simulink model "SPERTE_printer"  (R2026a)
settings: Solver=FixedStepDiscrete  StopTime=inf  FixedStep=Ts  EnableMultiTasking=on
InitFcn:
  | Fs = 1000; Ts = 1/Fs;tsim = Inf;
undefined symbols (not defined in the file or in its folder): DiscIntNeverNeededParam
libraries: simulink x11, sperte_lib x3
settings Model: SimulationMode=external  ExtModeTrigDuration=2  Creator=glife  LastModifiedBy=larsm
settings SolverCC: PositivePriorityOrder=on
settings OptimizationCC: PassReuseOutputArgsThreshold=0.0  MaxStackSize=200000
settings HardwareCC: ProdBitPerLong=64.0  ProdLargestAtomicInteger=LongLong  ProdLargestAtomicFloat=Double  ProdHWDeviceType=ARM Compatible->ARM Cortex-A (64-bit)  UseEmbeddedCoderFeatures=off
settings RTWCC: SystemTargetFile=ert.tlc  HardwareBoard=Raspberry Pi (64bit)  TLCOptions="-aInlineSetEventsForThisBaseRateFcn=TLC_FALSE -aSuppressMultiTaskScheduler=TLC_FALSE  -aRateBasedStepFcn=0"  PostCodeGenCommand="if (~verLessThan('matlab', '9.11')) codertarget.postCodeGenHookCommand(h);  SPERTE_postGenFunc(modelName, buildInfo); else; SPERTE_postGenFunc(h, buildInfo); end"  Toolchain=GNU GCC RPIUtils  BuildConfiguration=Faster Runs  Description=Embedded Coder
settings ERTTargetCC: ExtMode=on  ExtModeTransport=2.0  ExtModeMexArgs='131.155.56.35' 1 17725  ERTSrcFileBannerTemplate=codertarget_code_template.cgt  ERTHdrFileBannerTemplate=codertarget_code_template.cgt  ERTDataSrcFileTemplate=codertarget_code_template.cgt  ERTDataHdrFileTemplate=codertarget_code_template.cgt  DynamicArrayContainerType=coder::array  ERTCustomFileBanners=off  SupportContinuousTime=on  SupportNonInlinedSFcns=on  SupportVariableSizeSignals=on  ModelStepFunctionPrototypeControlCompliant=off

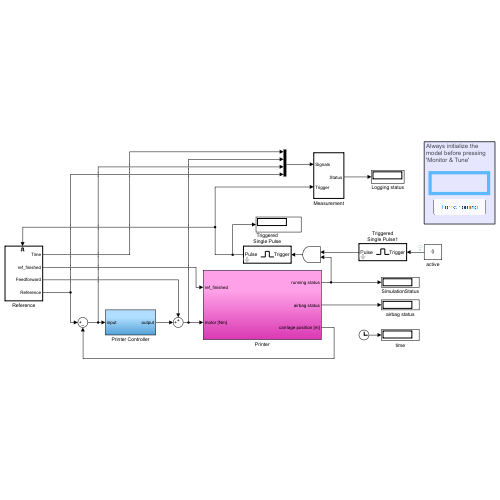
[thumbnail: Simulink's stored preview of the top-level diagram]
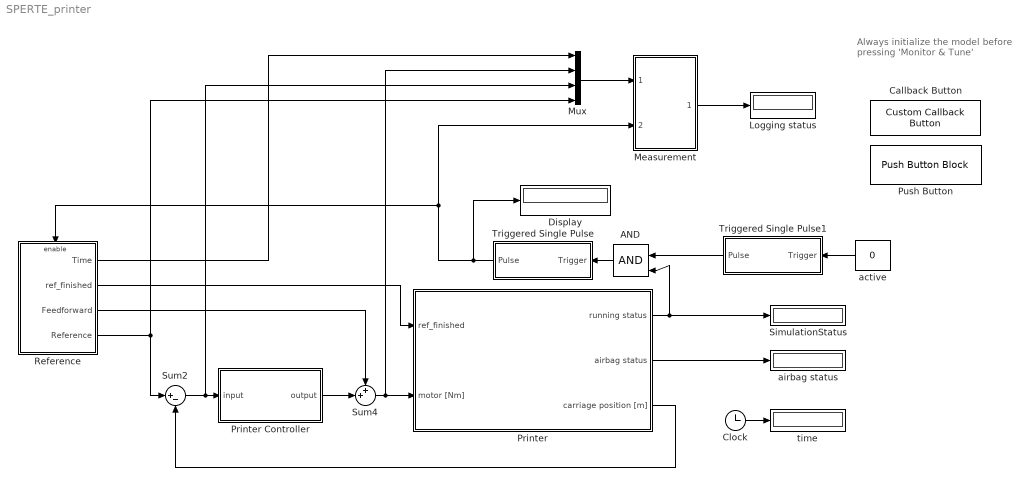
== system SPERTE_printer ==
  note: Always initialize the
      | model before pressing
      | 'Monitor & Tune'
  AND : Logic  IconShape=distinctive  AllPortsSameDT=off  OutDataTypeStr=boolean
  Callback Button : CustomCallbackButton  Configuration="{\"components\":[{\"name\":\"BackgroundImageComponent\",\"settings\":{\"image\":{\"size\":[0,0],\"src\":\"default\",\"srcOrientation\":\"Right\"},\"position\":[0,0,1,1]}},{\"name\":\"ButtonStateComponent\",\"settings\":{\"buttonType\":\"momentary\",\"clickFcn\":\"set_param('SPERTE_printer\\/Reference\\/set_Ref','Value','zeros(4501,1)');\\nset_param('SPERTE_printer\\/Reference\\/set_ff','Value','zeros(4501,1)');\\nset_param('SPERTE_printer\\/active','Value','0');\\nset_param('SPERTE_printer\\/Printer\\/force_home','Value','0');\\nmsgbox('Successfully initialized the model.');\",\"onValue\":1,\"position\":[0,0,1,1],\"pressDelay\":\"500\",\"pressFcn\":\"\",\"repeatInterval\":\"0\",\"states\":[{\"horizontalAlignment\":\"center\",\"image\":{\"position\":[0,0,1,1],\"src\":\"default\",\"srcOrientation\":\"Right\"},\"label\":{\"color\":[0.01176470588,0.01176470588,0.01176470588,1],\"icon\":{\"size\":[0,0],\"src\":\"default\",\"srcOrientation\":\"Right\"},\"iconPlacement\":\"left\",\"text\":{\"content\":\"INITIALIZE MODEL\"}},\"labelOffset\":[0,0],\"verticalAlignment\":\"middle\"},{\"horizontalAlignment\":\"center\",\"image\":{\"position\":[0,0,1,1],\"src\":\"default\",\"srcOrientation\":\"Right\"},\"label\":{\"color\":[0.01176470588,0.01176470588,0.01176470588,1],\"icon\":{\"size\":[0,0],\"src\":\"default\",\"srcOrientation\":\"Right\"},\"iconPlacement\":\"left\",\"text\":{\"content\":\"INITIALIZE MODEL\"}},\"labelOffset\":[0,0],\"verticalAlignment\":\"middle\"},{\"horizontalAlignment\":\"center\",\"image\":{\"position\":[0,0,1,1],\"src\":\"default\",\"srcOrientation\":\"Right\"},\"label\":{\"color\":[0.01176470588,0.01176470588,0.01176470588,1],\"icon\":{\"size\":[0,0],\"src\":\"default\",\"srcOrientation\":\"Right\"},\"iconPlacement\":\"left\",\"text\":{\"content\":\"INITIALIZE MODEL\"}},\"labelOffset\":[0,0],\"verticalAlignment\":\"middle\"},{\"horizontalAlignment\":\"center\",\"image\":{\"position\":[0,0,1,1],\"src\":\"default\",\"srcOrientation\":\"Right\"},\"label\":{\"color\":[0.01176470588,0.01176470588,0.01176470588,1],\"icon\":{\"size\":[0,0],\"src\":\"default\",\"srcOrientation\":\"Right\"},\"iconPlacement\":\"left\",\"text\":{\"content\":\"INITIALIZE MODEL\"}},\"labelOffset\":[0,0],\"verticalAlignment\":\"middle\"}]}},{\"name\":\"ForegroundImageComponent\",\"settings\":{\"image\":{\"size\":[0,0],\"src\":\"default\",\"srcOrientation\":\"Right\"},\"isForeground\":1,\"position\":[0,0,1,1]}}],\"derived\":{\"blockParameters\":{\"AutoActivate\":true,\"ButtonText\":\"INITIALIZE MODEL\",\"ButtonType\":\"Momentary\",\"ClickFcn\":\"set_param('SPERTE_printer\\/Reference\\/set_Ref','Value','zeros(4501,1)');\\nset_param('SPERTE_printer\\/Reference\\/set_ff','Value','zeros(4501,1)');\\nset_param('SPERTE_printer\\/active','Value','0');\\nset_param('SPERTE_printer\\/Printer\\/force_home','Value','0');\\nmsgbox('Successfully initialized the model.');\",\"OnValue\":1,\"PressDelay\":\"500\",\"PressFcn\":\"\",\"RepeatInterval\":\"0\",\"fixedAspectRatio\":\"off\"}},\"settings\":{\"BindingType\":\"standalone\",\"autoActivate\":true,\"backgroundColor\":[244,244,244,1],\"backgroundOffset\":0.2,\"backgroundOpacity\":1,\"fixedAspectRatio\":\"off\",\"foregroundColor\":[0.01176470588,0.01176470588,0.01176470588,1],\"migratedFromLegacy\":true,\"useBackgroundColor\":true,\"variant\":\"callback\",\"version\":\"R2024b\"},\"type\":\"Button\"}"  CustomBackgroundColor="{\"color\":[0.9568627451,0.9568627451,0.9568627451],\"show\":true}"
  Clock : Clock
  Display : Display
  Logging status : Display
  Measurement : Subsystem  TreatAsAtomicUnit=on
  Mux : Mux
  Printer : Subsystem
  Printer Controller : Subsystem
  Push Button : PushButtonBlock  ButtonText=Force homing  IconOnColor=[0.0, 0.39215686274509803, 0.0]  IconOffColor=[0.0, 1.0, 0.0]  OffValue=0.000000
  Reference : Subsystem  TreatAsAtomicUnit=on
  SimulationStatus : Display
      settings: Decimation=50
  Sum2 : Sum  Inputs=|+-
  Sum4 : Sum  Inputs=++|  InputSameDT=on  SaturateOnIntegerOverflow=on  OutDataTypeStr=Inherit: Same as first input
  Triggered Single Pulse : Subsystem  TreatAsAtomicUnit=on  mask(single pulse generation){p_wid=4502}
      mask prompts: p_wid "pulse width (number of samples)"
      mask help: This block generate a single pulse whenever a trigger happen. The pulse width must specified as a number of samples. for example if your sampling time is 0.1s and you want 3s pulse , then you should enter 30 as a pulse width.
      mask Display:
      | plot([0],[0])
      | plot([11],[0])
      | plot([5],[0.5])
      | plot([4 5 5 6 6 7],[0 0 0.25 0.25 0 0])
      | plot([5],[-0.3])
      | 
      | port_label('output', 1, 'Pulse')
      | port_label('input', 1, 'Trigger')
  Triggered Single Pulse1 : Subsystem  TreatAsAtomicUnit=on  mask(single pulse generation){p_wid=4502}
      mask prompts: p_wid "pulse width (number of samples)"
      mask help: This block generate a single pulse whenever a trigger happen. The pulse width must specified as a number of samples. for example if your sampling time is 0.1s and you want 3s pulse , then you should enter 30 as a pulse width.
      mask Display:
      | plot([0],[0])
      | plot([11],[0])
      | plot([5],[0.5])
      | plot([4 5 5 6 6 7],[0 0 0.25 0.25 0 0])
      | plot([5],[-0.3])
      | 
      | port_label('output', 1, 'Pulse')
      | port_label('input', 1, 'Trigger')
  active : Constant  Value=0
  airbag status : Display
      settings: Decimation=50
  time : Display
      settings: Decimation=50
  wires:
  Printer/3(carriage position [m]) -> Sum2/2
  Printer/2(airbag status) -> airbag status/1
  Sum2/1 -> Printer Controller/1(input), Mux/3
  Sum4/1 -> Printer/2(motor [Nm]), Mux/2
  Clock/1 -> time/1
  Printer Controller/1(output) -> Sum4/2
  AND/1 -> Triggered Single Pulse/1(Trigger)
  Reference/4(Reference) -> Sum2/1, Mux/4
  Reference/1(Time) -> Mux/1
  Mux/1 -> Measurement/1(Signals)
  Measurement/1(Status) -> Logging status/1
  Reference/3(Feedforward) -> Sum4/1
  Reference/2(ref_finished) -> Printer/1(ref_finished)
  Printer/1(running status) -> SimulationStatus/1, AND/2
  active/1 -> Triggered Single Pulse1/1(Trigger)
  Triggered Single Pulse/1(Pulse) -> Display/1, Measurement/2(Trigger), Reference/Enable
  Triggered Single Pulse1/1(Pulse) -> AND/1

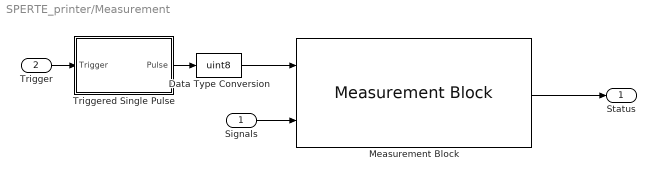
== system SPERTE_printer/Measurement ==
  Signals : Inport
  Trigger : Inport  Port=2
  Data Type Conversion : DataTypeConversion  OutDataTypeStr=uint8  SaturateOnIntegerOverflow=off  RndMeth=Floor
  Measurement Block : sperte_lib/Measurement/Measurement Block  Description=|  Priority=-1  N_samples=4501  triggertype=2  trigger_command=0
      | Perform on-demand measurements to file using this block.
      | 
      | It can be used in 2 ways:
      | 1) Set the mask triggertype parameter to manual and use the trigger input signal to trigger a measurement.
      | You can do this by providing a 0 to 1 transition.
      | Keep it low after you start/complete the measurement, or it will measure again.
      | A file is created with measurement_0,1,2... etc
      | 
      | 2) Keep the model running, and trigger a measurement from the commandline or Matlab script.
      | For example:
      | 
      | % How many samples to measure?
      | N_samples = Fs*5;
      | % Do the measurement
      | SPERTE_Perform_Measurement(N_samples);
      | % Get the latest file
      | file_list = SPERTE_Get_Latest_Measurement(p,1,'./data');
      | % How many signals did you record?
      | N_signals = 3;
      | % Convert the .bin to .mat and return the results
      | measurement = SPERTE_Bin_To_Mat(file_list,N_signals);
      settings: SourceProductName=SPERTE library
  Triggered Single Pulse : Subsystem  TreatAsAtomicUnit=on  mask(single pulse generation){p_wid=20}
      mask prompts: p_wid "pulse width (number of samples)"
      mask help: This block generate a single pulse whenever a trigger happen. The pulse width must specified as a number of samples. for example if your sampling time is 0.1s and you want 3s pulse , then you should enter 30 as a pulse width.
      mask Display:
      | plot([0],[0])
      | plot([11],[0])
      | plot([5],[0.5])
      | plot([4 5 5 6 6 7],[0 0 0.25 0.25 0 0])
      | plot([5],[-0.3])
      | 
      | port_label('output', 1, 'Pulse')
      | port_label('input', 1, 'Trigger')
  Status : Outport
  wires:
  Data Type Conversion/1 -> Measurement Block/1
  Measurement Block/1 -> Status/1
  Signals/1 -> Measurement Block/2
  Triggered Single Pulse/1(Pulse) -> Data Type Conversion/1
  Trigger/1 -> Triggered Single Pulse/1(Trigger)

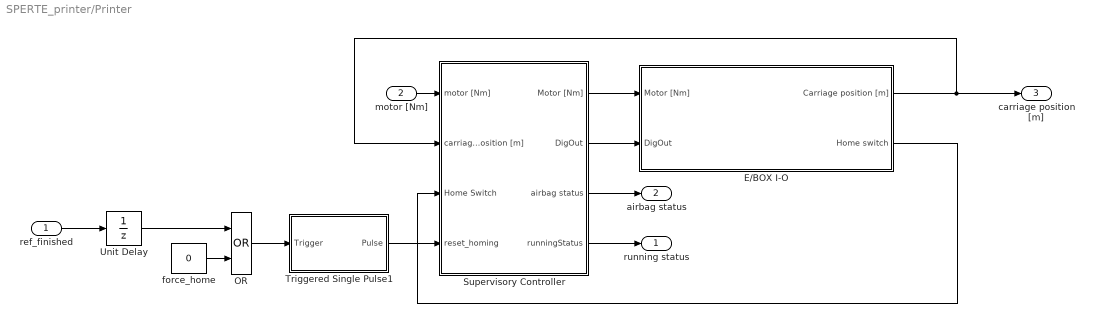
== system SPERTE_printer/Printer ==
  ref_finished : Inport
  motor [Nm] : Inport  Port=2
  E/BOX I-O : Subsystem
  OR : Logic  Operator=OR  IconShape=distinctive  AllPortsSameDT=off  OutDataTypeStr=boolean
  Supervisory Controller : Subsystem
  Triggered Single Pulse1 : Subsystem  TreatAsAtomicUnit=on  mask(single pulse generation){p_wid=1}
      mask prompts: p_wid "pulse width (number of samples)"
      mask help: This block generate a single pulse whenever a trigger happen. The pulse width must specified as a number of samples. for example if your sampling time is 0.1s and you want 3s pulse , then you should enter 30 as a pulse width.
      mask Display:
      | plot([0],[0])
      | plot([11],[0])
      | plot([5],[0.5])
      | plot([4 5 5 6 6 7],[0 0 0.25 0.25 0 0])
      | plot([5],[-0.3])
      | 
      | port_label('output', 1, 'Pulse')
      | port_label('input', 1, 'Trigger')
  Unit Delay : UnitDelay  SampleTime=-1
  force_home : Constant  Value=0
  running status : Outport
  airbag status : Outport  Port=2
  carriage position [m] : Outport  Port=3
  wires:
  E/BOX I-O/1(Carriage position [m]) -> Supervisory Controller/2(carriage position [m]), carriage position [m]/1
  Supervisory Controller/1(Motor [Nm]) -> E/BOX I-O/1(Motor [Nm])
  E/BOX I-O/2(Home switch) -> Supervisory Controller/3(Home Switch)
  motor [Nm]/1 -> Supervisory Controller/1(motor [Nm])
  Supervisory Controller/3(airbag status) -> airbag status/1
  Supervisory Controller/4(runningStatus) -> running status/1
  Supervisory Controller/2(DigOut) -> E/BOX I-O/2(DigOut)
  ref_finished/1 -> Unit Delay/1
  Triggered Single Pulse1/1(Pulse) -> Supervisory Controller/4(reset_homing)
  OR/1 -> Triggered Single Pulse1/1(Trigger)
  force_home/1 -> OR/2
  Unit Delay/1 -> OR/1

== system SPERTE_printer/Printer Controller ==
  input : Inport
  Dct2lowpass : S-Function  FunctionName=dlowpass2  Parameters=f_den, b_den, 0.001  SFunctionDeploymentMode=off  EnableBusSupport=off  mask(dctools){f_den=40, b_den=0.7}
      mask prompts: f_den "Pole [Hz]"; b_den "Damping pole [-]"
      mask help: This block implements a discrete time 2nd order lowpass filter.
      mask Display: disp('DCT 2nd order lowpass')
  Dctpd : S-Function  FunctionName=dpd  Parameters=kp, kv, 0.001  SFunctionDeploymentMode=off  EnableBusSupport=off  mask(dctools){kp=40, kv=1}
      mask help: This block implements a discrete time pd filter.
      mask Display: disp('DCT pd')
  Gain : Gain  Gain=4  SaturateOnIntegerOverflow=on  OutDataTypeStr=Inherit: Same as input  ParamDataTypeStr=Inherit: Same as input
  output : Outport
  wires:
  input/1 -> Gain/1
  Gain/1 -> Dctpd/1
  Dctpd/1 -> Dct2lowpass/1
  Dct2lowpass/1 -> output/1

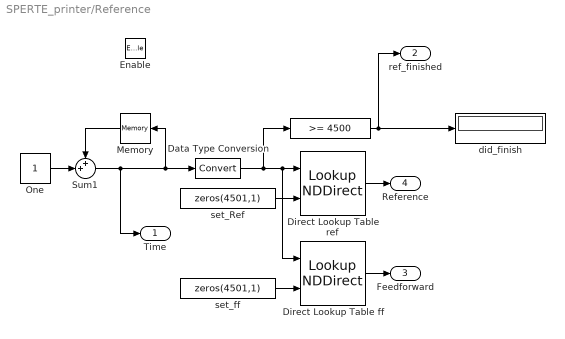
== system SPERTE_printer/Reference ==
  Enable : EnablePort  StatesWhenEnabling=reset
  " " : simulink/Logic and Bit Operations/Compare To Constant  relop=>=  const=4500  OutDataTypeStr=boolean
  Data Type Conversion : DataTypeConversion  SaturateOnIntegerOverflow=off  RndMeth=Floor
  Direct Lookup Table ff : LookupNDDirect  NumberOfTableDimensions=1  TableIsInput=on  Table=[4 5 ;16 19 ]  DiagnosticForOutOfRangeInput=Error
  Direct Lookup Table ref : LookupNDDirect  NumberOfTableDimensions=1  TableIsInput=on  Table=[4 5 ;16 19 ]  DiagnosticForOutOfRangeInput=Error
  Memory : Memory
  One : Constant  OutDataTypeStr=Inherit: Inherit via back propagation
  Sum1 : Sum  Inputs=++|
  did_finish : Display
  set_Ref : Constant  Value=zeros(4501,1)
  set_ff : Constant  Value=zeros(4501,1)
  Time : Outport
  ref_finished : Outport  Port=2
  Feedforward : Outport  Port=3
  Reference : Outport  Port=4
  wires:
  set_Ref/1 -> Direct Lookup Table ref/2
  Data Type Conversion/1 -> Direct Lookup Table ff/1, Direct Lookup Table ref/1, " "/1
  One/1 -> Sum1/2
  Direct Lookup Table ref/1 -> Reference/1
  Sum1/1 -> Data Type Conversion/1, Memory/1, Time/1
  Memory/1 -> Sum1/1
  Direct Lookup Table ff/1 -> Feedforward/1
  set_ff/1 -> Direct Lookup Table ff/2
  " "/1 -> did_finish/1, ref_finished/1

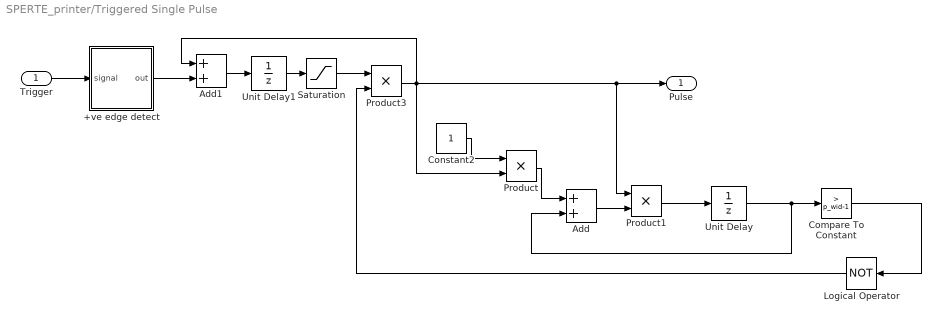
== system SPERTE_printer/Triggered Single Pulse ==
  Trigger : Inport
  +ve edge detect : Subsystem
  Add : Sum
  Add1 : Sum
  Compare To Constant : simulink/Logic and Bit Operations/Compare To Constant  relop=>  const=p_wid-1  OutDataTypeStr=boolean
  Constant2 : Constant
  Logical Operator : Logic  Operator=NOT  AllPortsSameDT=off  OutDataTypeStr=boolean
  Product : Product  RndMeth=Zero
  Product1 : Product  RndMeth=Zero
  Product3 : Product  RndMeth=Zero
  Saturation : Saturate  UpperLimit=1  LowerLimit=0
  Unit Delay : UnitDelay  SampleTime=-1
  Unit Delay1 : UnitDelay  SampleTime=-1
  Pulse : Outport
  wires:
  Compare To Constant/1 -> Logical Operator/1
  Constant2/1 -> Product/1
  Product/1 -> Add/1
  Unit Delay/1 -> Add/2, Compare To Constant/1
  Trigger/1 -> +ve edge detect/1(signal)
  +ve edge detect/1(out) -> Add1/2
  Add/1 -> Product1/2
  Product1/1 -> Unit Delay/1
  Add1/1 -> Unit Delay1/1
  Unit Delay1/1 -> Saturation/1
  Saturation/1 -> Product3/1
  Product3/1 -> Add1/1, Product/2, Product1/1, Pulse/1
  Logical Operator/1 -> Product3/2

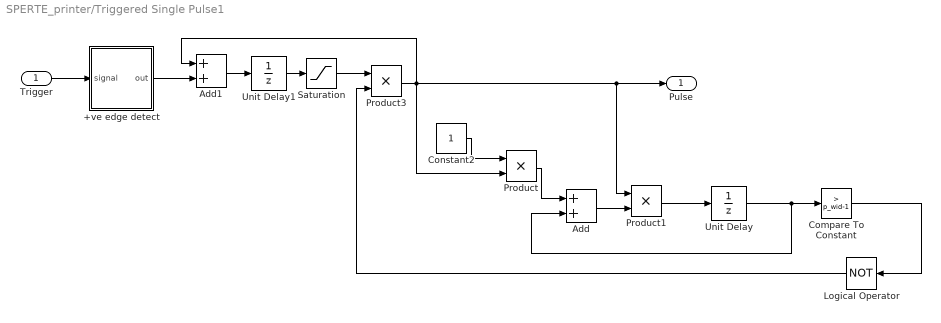
== system SPERTE_printer/Triggered Single Pulse1 ==
  Trigger : Inport
  +ve edge detect : Subsystem
  Add : Sum
  Add1 : Sum
  Compare To Constant : simulink/Logic and Bit Operations/Compare To Constant  relop=>  const=p_wid-1  OutDataTypeStr=boolean
  Constant2 : Constant
  Logical Operator : Logic  Operator=NOT  AllPortsSameDT=off  OutDataTypeStr=boolean
  Product : Product  RndMeth=Zero
  Product1 : Product  RndMeth=Zero
  Product3 : Product  RndMeth=Zero
  Saturation : Saturate  UpperLimit=1  LowerLimit=0
  Unit Delay : UnitDelay  SampleTime=-1
  Unit Delay1 : UnitDelay  SampleTime=-1
  Pulse : Outport
  wires:
  Compare To Constant/1 -> Logical Operator/1
  Constant2/1 -> Product/1
  Product/1 -> Add/1
  Unit Delay/1 -> Add/2, Compare To Constant/1
  Trigger/1 -> +ve edge detect/1(signal)
  +ve edge detect/1(out) -> Add1/2
  Add/1 -> Product1/2
  Product1/1 -> Unit Delay/1
  Add1/1 -> Unit Delay1/1
  Unit Delay1/1 -> Saturation/1
  Saturation/1 -> Product3/1
  Product3/1 -> Add1/1, Product/2, Product1/1, Pulse/1
  Logical Operator/1 -> Product3/2

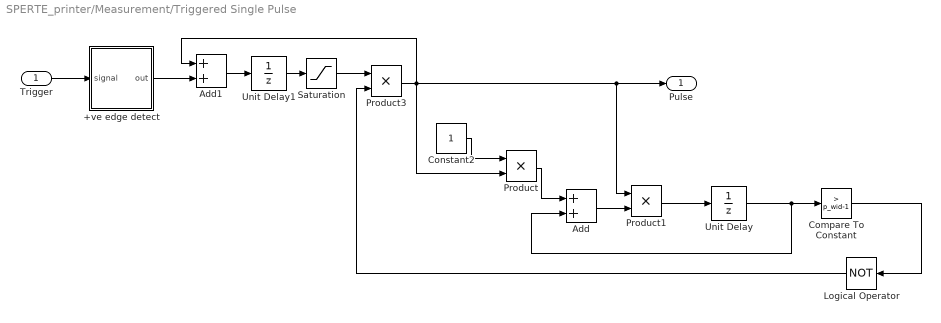
== system SPERTE_printer/Measurement/Triggered Single Pulse ==
  Trigger : Inport
  +ve edge detect : Subsystem
  Add : Sum
  Add1 : Sum
  Compare To Constant : simulink/Logic and Bit Operations/Compare To Constant  relop=>  const=p_wid-1  OutDataTypeStr=boolean
  Constant2 : Constant
  Logical Operator : Logic  Operator=NOT  AllPortsSameDT=off  OutDataTypeStr=boolean
  Product : Product  RndMeth=Zero
  Product1 : Product  RndMeth=Zero
  Product3 : Product  RndMeth=Zero
  Saturation : Saturate  UpperLimit=1  LowerLimit=0
  Unit Delay : UnitDelay  SampleTime=-1
  Unit Delay1 : UnitDelay  SampleTime=-1
  Pulse : Outport
  wires:
  Compare To Constant/1 -> Logical Operator/1
  Constant2/1 -> Product/1
  Product/1 -> Add/1
  Unit Delay/1 -> Add/2, Compare To Constant/1
  Trigger/1 -> +ve edge detect/1(signal)
  +ve edge detect/1(out) -> Add1/2
  Add/1 -> Product1/2
  Product1/1 -> Unit Delay/1
  Add1/1 -> Unit Delay1/1
  Unit Delay1/1 -> Saturation/1
  Saturation/1 -> Product3/1
  Product3/1 -> Add1/1, Product/2, Product1/1, Pulse/1
  Logical Operator/1 -> Product3/2

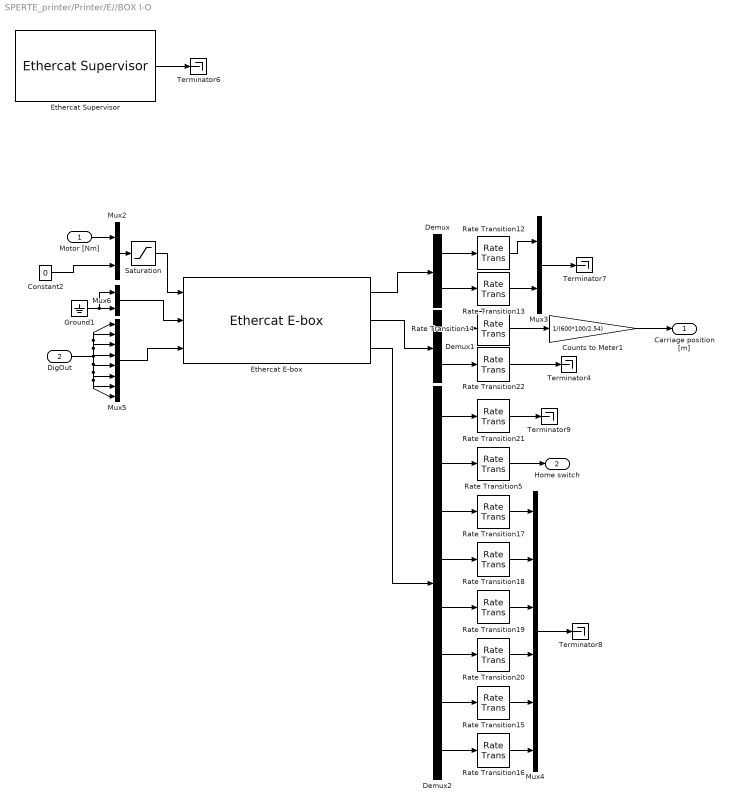
== system SPERTE_printer/Printer/E//BOX I-O ==
  Motor [Nm] : Inport
  DigOut : Inport  Port=2
  Constant2 : Constant  Value=0
  Counts to Meter1 : Gain  Gain=1/(600*100/2.54)
  Demux : Demux  Outputs=2
  Demux1 : Demux  Outputs=2
  Demux2 : Demux  Outputs=8
  Ethercat E-box : sperte_lib/EtherCAT/Ethercat E-box  Priority=-2  link_id=0
      settings: SourceProductName=SPERTE library
  Ethercat Supervisor : sperte_lib/EtherCAT/Ethercat Supervisor  Description=Must be executed first, keep at -1 priority (highest)  Priority=-3  portid=0  ectimeout=500
      settings: SourceProductName=SPERTE library
  Ground1 : Ground
  Mux2 : Mux  Inputs=2
  Mux3 : Mux  Inputs=2
  Mux4 : Mux  Inputs=6
  Mux5 : Mux  Inputs=8
  Mux6 : Mux  Inputs=2
  Rate Transition{5,12..22} (12 alike) : RateTransition
  Saturation : Saturate  UpperLimit=2.5  LowerLimit=-2.5
  Terminator{4,6..9} (5 alike) : Terminator
  Carriage position [m] : Outport
  Home switch : Outport  Port=2
  wires:
  Motor [Nm]/1 -> Mux2/1
  Demux2/2 -> Rate Transition5/1
  Rate Transition5/1 -> Home switch/1
  Saturation/1 -> Ethercat E-box/1
  Ethercat E-box/3 -> Demux2/1
  Ground1/1 -> Mux6/1, Mux6/2
  Ethercat Supervisor/1 -> Terminator6/1
  Ethercat E-box/2 -> Demux1/1
  Constant2/1 -> Mux2/2
  Mux2/1 -> Saturation/1
  Counts to Meter1/1 -> Carriage position [m]/1
  Ethercat E-box/1 -> Demux/1
  Demux/1 -> Rate Transition12/1
  Demux/2 -> Rate Transition13/1
  Rate Transition13/1 -> Mux3/2
  Mux3/1 -> Terminator7/1
  Rate Transition12/1 -> Mux3/1
  Rate Transition14/1 -> Counts to Meter1/1
  Demux1/1 -> Rate Transition14/1
  Demux1/2 -> Rate Transition22/1
  Rate Transition19/1 -> Mux4/3
  Rate Transition18/1 -> Mux4/2
  Rate Transition20/1 -> Mux4/4
  Demux2/8 -> Rate Transition16/1
  Rate Transition17/1 -> Mux4/1
  Demux2/5 -> Rate Transition19/1
  Demux2/6 -> Rate Transition20/1
  Demux2/4 -> Rate Transition18/1
  Rate Transition15/1 -> Mux4/5
  Mux4/1 -> Terminator8/1
  Demux2/3 -> Rate Transition17/1
  Demux2/7 -> Rate Transition15/1
  Rate Transition16/1 -> Mux4/6
  Rate Transition21/1 -> Terminator9/1
  Demux2/1 -> Rate Transition21/1
  Mux5/1 -> Ethercat E-box/3
  DigOut/1 -> Mux5/8, Mux5/7, Mux5/6, Mux5/5, Mux5/4, Mux5/1, Mux5/2, Mux5/3
  Mux6/1 -> Ethercat E-box/2
  Rate Transition22/1 -> Terminator4/1

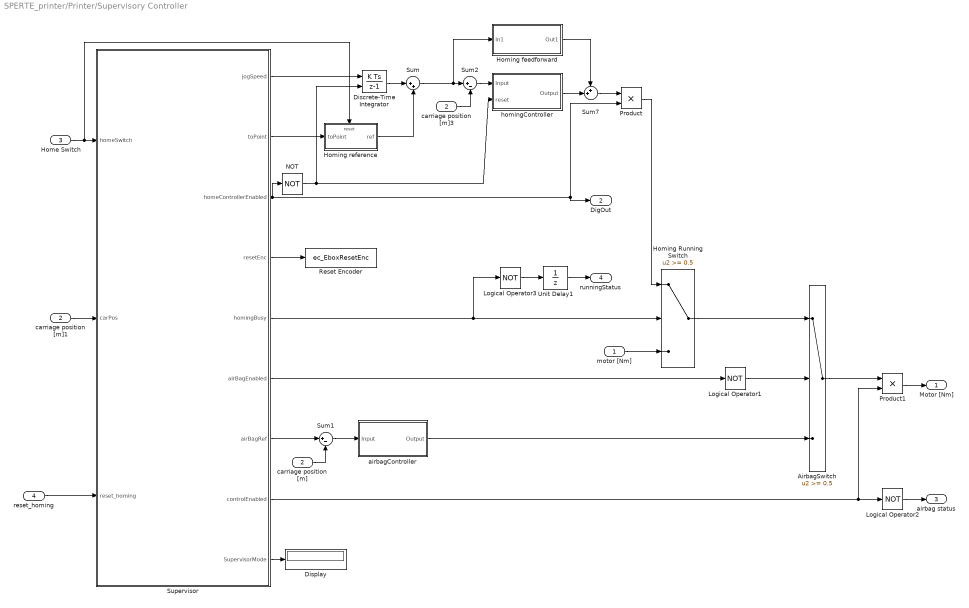
== system SPERTE_printer/Printer/Supervisory Controller ==
  motor [Nm] : Inport
  carriage position [m] : Inport  Port=2
  Home Switch : Inport  Port=3
  reset_homing : Inport  Port=4
  AirbagSwitch : Switch  Threshold=0.5  SaturateOnIntegerOverflow=off  InputSameDT=off
  Discrete-Time Integrator : DiscreteIntegrator  ExternalReset=level  SampleTime=-1  ICPrevOutput=DiscIntNeverNeededParam  ICPrevScaledInput=DiscIntNeverNeededParam
  Display : Display
  Homing Running Switch : Switch  Threshold=0.5  SaturateOnIntegerOverflow=off  InputSameDT=off
  Homing feedforward : Subsystem
  Homing reference : Subsystem
  Logical Operator1 : Logic  Operator=NOT  AllPortsSameDT=off  OutDataTypeStr=boolean
  Logical Operator2 : Logic  Operator=NOT  AllPortsSameDT=off  OutDataTypeStr=boolean
  Logical Operator3 : Logic  Operator=NOT  AllPortsSameDT=off  OutDataTypeStr=boolean
  NOT : Logic  Operator=NOT  IconShape=distinctive  AllPortsSameDT=off  OutDataTypeStr=boolean
  Product : Product  RndMeth=Zero
  Product1 : Product  RndMeth=Zero
  Reset Encoder : S-Function  FunctionName=ec_EboxResetEnc  Parameters=link_id  SFunctionDeploymentMode=off  EnableBusSupport=off  mask{link_id=0}
      mask prompts: link_id "analog in id (start from 1)"
  Sum : Sum  Inputs=|++
  Sum1 : Sum  Inputs=|+-
  Sum2 : Sum  Inputs=|+-
  Sum7 : Sum  Inputs=++|
  Supervisor : Stateflow chart  TreatAsAtomicUnit=on
  Unit Delay1 : UnitDelay  SampleTime=-1
  airbagController : Subsystem
  carriage position [m]1 : InportShadow  Port=2
  carriage position [m]3 : InportShadow  Port=2
  homingController : Subsystem
  Motor [Nm] : Outport
  DigOut : Outport  Port=2
  airbag status : Outport  Port=3
  runningStatus : Outport  Port=4
  wires:
  Homing Running Switch/1 -> AirbagSwitch/1
  Sum/1 -> Homing feedforward/1(In1), Sum2/1
  Sum2/1 -> homingController/1(Input)
  Home Switch/1 -> Homing reference/Reset, Supervisor/1(homeSwitch)
  Supervisor/1(jogSpeed) -> Discrete-Time Integrator/1
  carriage position [m]3/1 -> Sum2/2
  motor [Nm]/1 -> Homing Running Switch/3
  homingController/1(Output) -> Sum7/2
  Product/1 -> Homing Running Switch/1
  Discrete-Time Integrator/1 -> Sum/1
  Supervisor/5(homingBusy) -> Homing Running Switch/2, Logical Operator3/1
  Supervisor/3(homeControllerEnabled) -> Product/2, DigOut/1, NOT/1
  Supervisor/2(toPoint) -> Homing reference/1(toPoint)
  Supervisor/4(resetEnc) -> Reset Encoder/1
  carriage position [m]1/1 -> Supervisor/2(carPos)
  Supervisor/6(airBagEnabled) -> Logical Operator1/1
  Logical Operator1/1 -> AirbagSwitch/2
  airbagController/1(Output) -> AirbagSwitch/3
  Sum1/1 -> airbagController/1(Input)
  carriage position [m]/1 -> Sum1/2
  Supervisor/7(airBagRef) -> Sum1/1
  AirbagSwitch/1 -> Product1/1
  Product1/1 -> Motor [Nm]/1
  Supervisor/8(controlEnabled) -> Logical Operator2/1, Product1/2
  Logical Operator2/1 -> airbag status/1
  Logical Operator3/1 -> Unit Delay1/1
  Supervisor/9(SupervisorMode) -> Display/1
  Unit Delay1/1 -> runningStatus/1
  reset_homing/1 -> Supervisor/3(reset_homing)
  NOT/1 -> homingController/2(reset), Discrete-Time Integrator/2
  Sum7/1 -> Product/1
  Homing reference/1(ref) -> Sum/2
  Homing feedforward/1(Out1) -> Sum7/1

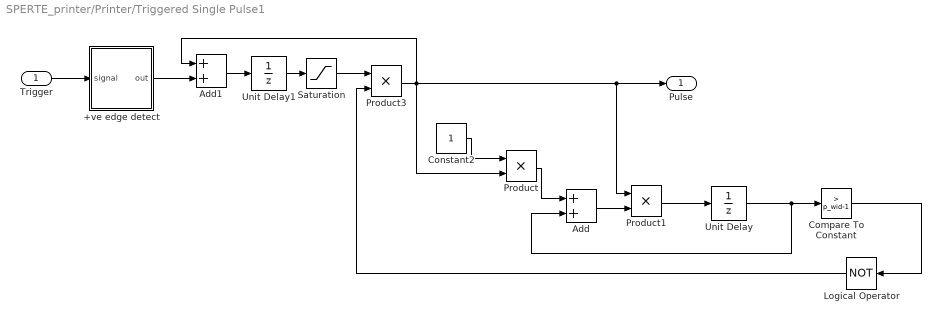
== system SPERTE_printer/Printer/Triggered Single Pulse1 ==
  Trigger : Inport
  +ve edge detect : Subsystem
  Add : Sum
  Add1 : Sum
  Compare To Constant : simulink/Logic and Bit Operations/Compare To Constant  relop=>  const=p_wid-1  OutDataTypeStr=boolean
  Constant2 : Constant
  Logical Operator : Logic  Operator=NOT  AllPortsSameDT=off  OutDataTypeStr=boolean
  Product : Product  RndMeth=Zero
  Product1 : Product  RndMeth=Zero
  Product3 : Product  RndMeth=Zero
  Saturation : Saturate  UpperLimit=1  LowerLimit=0
  Unit Delay : UnitDelay  SampleTime=-1
  Unit Delay1 : UnitDelay  SampleTime=-1
  Pulse : Outport
  wires:
  Compare To Constant/1 -> Logical Operator/1
  Constant2/1 -> Product/1
  Product/1 -> Add/1
  Unit Delay/1 -> Add/2, Compare To Constant/1
  Trigger/1 -> +ve edge detect/1(signal)
  +ve edge detect/1(out) -> Add1/2
  Add/1 -> Product1/2
  Product1/1 -> Unit Delay/1
  Add1/1 -> Unit Delay1/1
  Unit Delay1/1 -> Saturation/1
  Saturation/1 -> Product3/1
  Product3/1 -> Add1/1, Product/2, Product1/1, Pulse/1
  Logical Operator/1 -> Product3/2

== system SPERTE_printer/Triggered Single Pulse/+ve edge detect ==
  note: Edge
  signal : Inport
  Delay Input1 : UnitDelay  Description=Store in Global RAM  DisableCoverage=on  SampleTime=-1
  FixPt Relational Operator : RelationalOperator  Operator=>  OutDataTypeStr=fixdt(0, 8)  ZeroCross=off  InputSameDT=off
  Positive : simulink/Logic and Bit Operations/Compare To Zero  relop=>  OutDataTypeStr=uint8  ZeroCross=off
  out : Outport
  wires:
  Delay Input1/1 -> FixPt Relational Operator/2  "U(k-1)"
  Positive/1 -> Delay Input1/1, FixPt Relational Operator/1  "U(k)"
  FixPt Relational Operator/1 -> out/1
  signal/1 -> Positive/1

== system SPERTE_printer/Triggered Single Pulse1/+ve edge detect ==
  note: Edge
  signal : Inport
  Delay Input1 : UnitDelay  Description=Store in Global RAM  DisableCoverage=on  SampleTime=-1
  FixPt Relational Operator : RelationalOperator  Operator=>  OutDataTypeStr=fixdt(0, 8)  ZeroCross=off  InputSameDT=off
  Positive : simulink/Logic and Bit Operations/Compare To Zero  relop=>  OutDataTypeStr=uint8  ZeroCross=off
  out : Outport
  wires:
  Delay Input1/1 -> FixPt Relational Operator/2  "U(k-1)"
  Positive/1 -> Delay Input1/1, FixPt Relational Operator/1  "U(k)"
  FixPt Relational Operator/1 -> out/1
  signal/1 -> Positive/1

== system SPERTE_printer/Measurement/Triggered Single Pulse/+ve edge detect ==
  note: Edge
  signal : Inport
  Delay Input1 : UnitDelay  Description=Store in Global RAM  DisableCoverage=on  SampleTime=-1
  FixPt Relational Operator : RelationalOperator  Operator=>  OutDataTypeStr=fixdt(0, 8)  ZeroCross=off  InputSameDT=off
  Positive : simulink/Logic and Bit Operations/Compare To Zero  relop=>  OutDataTypeStr=uint8  ZeroCross=off
  out : Outport
  wires:
  Delay Input1/1 -> FixPt Relational Operator/2  "U(k-1)"
  Positive/1 -> Delay Input1/1, FixPt Relational Operator/1  "U(k)"
  FixPt Relational Operator/1 -> out/1
  signal/1 -> Positive/1

== system SPERTE_printer/Printer/Supervisory Controller/Homing feedforward ==
  In1 : Inport
  Compare To Constant : simulink/Logic and Bit Operations/Compare To Constant  relop=>  const=0  OutDataTypeStr=uint8
  Discrete Derivative : simulink/Discrete/Discrete Derivative  gainval=1.0  ICPrevScaledInput=0.0  OutMin=[]  OutMax=[]  OutDataType=fixdt(1, 16)  OutScaling=2^-10  DoSatur=off
  Sign : Signum
  sign(v) BF : Gain  Gain=1.1342
  Out1 : Outport
  wires:
  In1/1 -> Discrete Derivative/1
  Discrete Derivative/1 -> Sign/1
  Sign/1 -> Compare To Constant/1
  Compare To Constant/1 -> sign(v) BF/1
  sign(v) BF/1 -> Out1/1

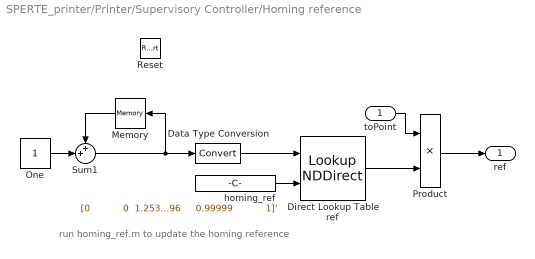
== system SPERTE_printer/Printer/Supervisory Controller/Homing reference ==
  note: run homing_ref.m to update the homing reference
  toPoint : Inport
  Reset : ResetPort  DisableCoverage=on
  Data Type Conversion : DataTypeConversion  SaturateOnIntegerOverflow=off  RndMeth=Floor
  Direct Lookup Table ref : LookupNDDirect  NumberOfTableDimensions=1  TableIsInput=on  Table=[4 5 ;16 19 ]  DiagnosticForOutOfRangeInput=Error
  Memory : Memory
  One : Constant  OutDataTypeStr=Inherit: Inherit via back propagation
  Product : Product  OutDataTypeStr=double
  Sum1 : Sum  Inputs=++|
  homing_ref : Constant  Value="[0           0  1.2531e-05  3.7594e-05  7.5188e-05  0.00012531  0.00018797  0.00026316  0.00035088  0.00045113  0.00056391  0.00068922  0.00082707  0.00097744   0.0011404   0.0013158   0.0015038   0.0017043   0.0019173   0.0021429    0.002381   0.0026316   0.0028947   0.0031704   0.0034586   0.0037594   0.0040727   0.0043985   0.0047368   0.0050877   0.0054511   0.0058271   0.0062155   0.0066165   0.0070301   0.0074561   0.0078947   0.0083459   0.0088095   0.0092857   0.0097744    0.010276    0.010789    0.011316    0.011855    0.012406     0.01297    0.013546    0.014135    0.014737    0.015351    0.015977    0.016617    0.017268    0.017932    0.018609    0.019298        0.02    0.020714    0.021441     0.02218    0.022932    0.023697    0.024474    0.025263    0.026065     0.02688    0.027707    0.028546    0.029398    0.030263     0.03114     0.03203    0.032932    0.033847    0.034774    0.035714    0.036667    0.037632    0.038609    0.039599    0.040602    0.041617    0.042644    0.043684    0.044737    0.045802     0.04688     0.04797    0.049073    0.050188    0.051316    0.052456    0.053609    0.054774    0.055952    0.057143    0.058346    0.059561    0.060789     0.06203    0.063283    0.064549    0.065827    0.067118    0.068421    0.069737    0.071065    0.072406    0.073759    0.075125    0.076504    0.077895    0.079298    0.080714    0.082143    0.083584    0.085038    0.086504    0.087982    0.089474    0.090977    0.092494    0.094023    0.095564    0.097118    0.098684     0.10026     0.10185     0.10346     0.10508      0.1067     0.10835        0.11     0.11167     0.11335     0.11504     0.11674     0.11846     0.12019     0.12193     0.12368     0.12545     0.12723     0.12902     0.13083     0.13264     0.13447     0.13632     0.13817     0.14004     0.14192     0.14381     0.14571     0.14763     0.14956      0.1515     0.15346     0.15543     0.15741      0.1594      0.1614     0.16342     0.16545     0.16749     0.16955     0.17162      0.1737     0.17579     0.17789     0.18001     0.18214     0.18429     0.18644     0.18861     0.19079     0.19298     0.19519     0.19741     0.19964     0.20188     0.20414      0.2064     0.20868     0.21098     0.21328      0.2156     0.21793     0.22028     0.22263       0.225     0.22738     0.22977     0.23218      0.2346     0.23703     0.23947     0.24193      0.2444     0.24688     0.24937     0.25188     0.25439     0.25689      0.2594      0.2619     0.26441     0.26692     0.26942     0.27193     0.27444     0.27694     0.27945     0.28195     0.28446     0.28697     0.28947     0.29198     0.29449     0.29699      0.2995     0.30201     0.30451     0.30702     0.30952     0.31203     0.31454     0.31704     0.31955     0.32206     0.32456     0.32707     0.32957     0.33208     0.33459     0.33709      0.3396     0.34211     0.34461     0.34712     0.34962     0.35213     0.35464     0.35714     0.35965     0.36216     0.36466     0.36717     0.36967     0.37218     0.37469     0.37719      0.3797     0.38221     0.38471     0.38722     0.38972     0.39223     0.39474     0.39724     0.39975     0.40226     0.40476     0.40727     0.40977     0.41228     0.41479     0.41729      0.4198     0.42231     0.42481     0.42732     0.42982     0.43233     0.43484     0.43734     0.43985     0.44236     0.44486     0.44737     0.44987     0.45238     0.45489     0.45739      0.4599     0.46241     0.46491     0.46742     0.46992     0.47243     0.47494     0.47744     0.47995     0.48246     0.48496     0.48747     0.48997     0.49248     0.49499     0.49749         0.5     0.50251     0.50501     0.50752     0.51003     0.51253     0.51504     0.51754     0.52005     0.52256     0.52506     0.52757     0.53008     0.53258     0.53509     0.53759      0.5401     0.54261     0.54511     0.54762     0.55013     0.55263     0.55514     0.55764     0.56015     0.56266     0.56516     0.56767     0.57018     0.57268     0.57519     0.57769      0.5802     0.58271 ...(+3191 chars)]'"
  ref : Outport
  wires:
  toPoint/1 -> Product/1
  Direct Lookup Table ref/1 -> Product/2
  Product/1 -> ref/1
  homing_ref/1 -> Direct Lookup Table ref/2
  Memory/1 -> Sum1/1
  One/1 -> Sum1/2
  Data Type Conversion/1 -> Direct Lookup Table ref/1
  Sum1/1 -> Data Type Conversion/1, Memory/1

== system SPERTE_printer/Printer/Supervisory Controller/airbagController ==
  Input : Inport
  Dct2lowpass3 : S-Function  FunctionName=dlowpass2  Parameters=f_den, b_den, 0.001  SFunctionDeploymentMode=off  EnableBusSupport=off  mask(dctools){f_den=40, b_den=0.7}
      mask prompts: f_den "Pole [Hz]"; b_den "Damping pole [-]"
      mask help: This block implements a discrete time 2nd order lowpass filter.
      mask Display: disp('DCT 2nd order lowpass')
  Dctpd2 : S-Function  FunctionName=dpd  Parameters=kp, kv, 0.001  SFunctionDeploymentMode=off  EnableBusSupport=off  mask(dctools){kp=40, kv=1}
      mask help: This block implements a discrete time pd filter.
      mask Display: disp('DCT pd')
  Gain1 : Gain  Gain=4  SaturateOnIntegerOverflow=on  OutDataTypeStr=Inherit: Same as input  ParamDataTypeStr=Inherit: Same as input
  Output : Outport
  wires:
  Input/1 -> Gain1/1
  Gain1/1 -> Dctpd2/1
  Dctpd2/1 -> Dct2lowpass3/1
  Dct2lowpass3/1 -> Output/1

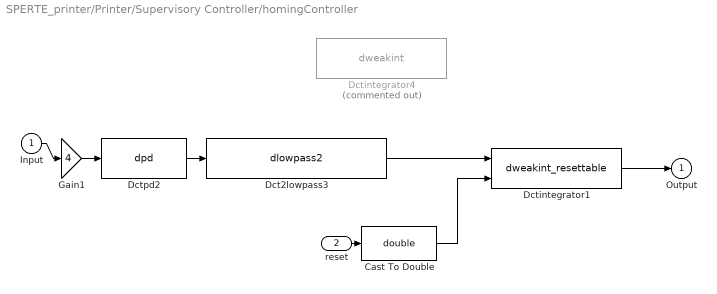
== system SPERTE_printer/Printer/Supervisory Controller/homingController ==
  Input : Inport
  reset : Inport  Port=2
  Cast To Double : DataTypeConversion  OutDataTypeStr=double  SaturateOnIntegerOverflow=off  RndMeth=Floor
  Dct2lowpass3 : S-Function  FunctionName=dlowpass2  Parameters=f_den, b_den, 0.001  SFunctionDeploymentMode=off  EnableBusSupport=off  mask(dctools){f_den=40, b_den=0.7}
      mask prompts: f_den "Pole [Hz]"; b_den "Damping pole [-]"
      mask help: This block implements a discrete time 2nd order lowpass filter.
      mask Display: disp('DCT 2nd order lowpass')
  Dctintegrator1 : S-Function  FunctionName=dweakint_resettable  Parameters=f_num, 0.001  SFunctionDeploymentMode=off  EnableBusSupport=off  mask(dctools){f_num=0.25}
      mask prompts: f_num "Zero [Hz]"
      mask help: This block implements a discrete time weak integrator filter.
      mask Display: disp('DCT integrator')
  Dctintegrator4 : S-Function  Commented=on  FunctionName=dweakint  Parameters=f_num, 0.001  SFunctionDeploymentMode=off  EnableBusSupport=off  mask(dctools){f_num=0.25}
      mask prompts: f_num "Zero [Hz]"
      mask help: This block implements a discrete time weak integrator filter.
      mask Display: disp('DCT integrator')
  Dctpd2 : S-Function  FunctionName=dpd  Parameters=kp, kv, 0.001  SFunctionDeploymentMode=off  EnableBusSupport=off  mask(dctools){kp=40, kv=1}
      mask help: This block implements a discrete time pd filter.
      mask Display: disp('DCT pd')
  Gain1 : Gain  Gain=4  SaturateOnIntegerOverflow=on  OutDataTypeStr=Inherit: Same as input  ParamDataTypeStr=Inherit: Same as input
  Output : Outport
  wires:
  Input/1 -> Gain1/1
  Gain1/1 -> Dctpd2/1
  Dctpd2/1 -> Dct2lowpass3/1
  Dctintegrator1/1 -> Output/1
  Cast To Double/1 -> Dctintegrator1/2
  Dct2lowpass3/1 -> Dctintegrator1/1
  reset/1 -> Cast To Double/1

== system SPERTE_printer/Printer/Triggered Single Pulse1/+ve edge detect ==
  note: Edge
  signal : Inport
  Delay Input1 : UnitDelay  Description=Store in Global RAM  DisableCoverage=on  SampleTime=-1
  FixPt Relational Operator : RelationalOperator  Operator=>  OutDataTypeStr=fixdt(0, 8)  ZeroCross=off  InputSameDT=off
  Positive : simulink/Logic and Bit Operations/Compare To Zero  relop=>  OutDataTypeStr=uint8  ZeroCross=off
  out : Outport
  wires:
  Delay Input1/1 -> FixPt Relational Operator/2  "U(k-1)"
  Positive/1 -> Delay Input1/1, FixPt Relational Operator/1  "U(k)"
  FixPt Relational Operator/1 -> out/1
  signal/1 -> Positive/1

== stateflow chart SPERTE_printer/Printer/Supervisory Controller/Supervisor ==
  state AirbagLeft
    entry:
    airBagEnabled = 1;
    airBagRef=-0.01;
  state DisableOutputs
    entry:
    controlEnabled=0;
  state Homing
    entry:
    %Set jog speed and homing state
    toPoint = 0;
    homingBusy = 1;
    jogSpeed = -0.2;
    homeControllerEnabled=1;
  state AirbagRight
    entry:
    airBagEnabled = 1;
    airBagRef=0.35;
  state EnableRunAndSafety
    entry:
    resetEnc=0;
    homingBusy=0;
  state MovetoX0
    entry:
    jogSpeed = 0.0;
    toPoint = 0.06;
  state ResetEnc
    entry:
    resetEnc=1;
  state DisableControl
    entry:
    homeControllerEnabled=0;
  (default) -> Homing
  AirbagLeft -> DisableOutputs : after(1,sec)
  AirbagRight -> DisableOutputs : after(1,sec)
  EnableRunAndSafety -> Homing [order 1] : [reset_homing]
  EnableRunAndSafety -> AirbagLeft [order 2] : [carPos<-0.01]
  Homing -> MovetoX0 : %Transition if homeswitch becomes high
      | [homeSwitch]
  EnableRunAndSafety -> AirbagRight [order 3] : [carPos>0.35]
  ResetEnc -> EnableRunAndSafety : after(0.1,sec)
  MovetoX0 -> DisableControl : %Allow time for moving
      | after(1,sec)
  DisableControl -> ResetEnc : %Allow settling of belt
      | after(0.5,sec)
  data: jogSpeed output double; toPoint output double; homeControllerEnabled output double; resetEnc output double; homingBusy output double =1; homeSwitch input double; carPos input double; airBagEnabled output double =0; airBagRef output double =0; controlEnabled output double =1; reset_homing input; SupervisorMode output Enum: SupervisorModeType
